simulink model "model"  (R2019b)
settings: Solver=VariableStepAuto  StartTime=0.0  StopTime=nb_time_unit_in_a_simulation/5  RelTol=1e-3
undefined symbols (not defined in the file or in its folder): air_mass_kg_rooms, Area_boiler, area_outdoor_rooms, Area_radiators, area_rooms_ground, area_walls_between_rooms, C_air, C_water, Energy_used_by_air_conditioner_for_1_timeunit_in_Watts_vector, Energy_used_by_air_mixer_for_1_timeunit_in_Watts, Energy_used_by_boiler_for_1_timeunit_in_Watts, initial_relative_humidity, initial_temp_water_in_boilers, initial_temperature_rooms, initial_temperature_water_in_radiator, k_boiler_border, k_radiators, k_wall_outdoor_rooms, k_walls_between_rooms, mass_water_radiator, matrix_AC_rooms_locations, matrix_boiler_radiator_connection, matrix_boiler_rooms_locations, matrix_radiator_rooms_locations, nb_air_cons, nb_boilers, nb_humans, nb_radiators, nb_rooms, nb_second_in_timeunit, outdoor_max_temp_A, outdoor_max_temp_B, outdoor_min_temp_A, outdoor_min_temp_B, tau_boiler, thickness_boiler, thickness_outdoor_rooms, thickness_radiator_pipes, thickness_walls_between_rooms, timeunit_in_a_day, Volume_radiators, Volume_rooms, water_weight_in_boiler, watt_generation_of_employe
libraries: dspmtrx3 x15, simulink x14
(part 2 of 2)

== system model/Physical model/Wall heat Exchange module/Value heat exchange outdoor -> rooms ==
  T_rooms : Inport
  outdoor : Inport  Port=2
  Gain : Gain  Gain=area_outdoor_rooms
  Gain1 : Gain  Gain=k_wall_outdoor_rooms
  Gain2 : Gain  Gain=ones(nb_rooms,1)./thickness_outdoor_rooms
  Sum : Sum  Inputs=|+-
  Q_outdoor_to_rooms : Outport
  wires:
  T_rooms/1 -> Sum/2
  outdoor/1 -> Sum/1
  Sum/1 -> Gain/1
  Gain/1 -> Gain1/1
  Gain1/1 -> Gain2/1
  Gain2/1 -> Q_outdoor_to_rooms/1

== system model/Physical model/Wall heat Exchange module/Value heat exchange within building ==
  "T_rooms " : Inport
  Constant : Constant  Value=diag(ones(nb_rooms,1))
  Gain3 : Gain  Gain=area_walls_between_rooms
  Gain4 : Gain  Gain=k_walls_between_rooms
  Gain8 : Gain  Gain=ones(nb_rooms,nb_rooms)./thickness_walls_between_rooms
  MATRIX WITH ROOM TEMPERATURE DIFFERENCE The area matrix after handles the case of non-adjacent rooms : dspmtrx3/Array-Vector Multiply  mode=Mute  saveAsFlag=0  Dimension=2  V_Source=Input port  V_VectFromMask=[0.5 0.25]  roundingMode=Floor  overflowMode=off  firstCoeffSignedness=Auto  firstCoeffDataTypeStr=Inherit: Same word length as input  firstCoeffMin=[]  firstCoeffMax=[]  firstCoeffLastDataTypeStr=Inherit: Same word length as input  prodOutputSignedness=Auto  accumSignedness=Auto  outputSignedness=Auto  outputDataTypeStr=Inherit: Same as product output  outputMin=[]  outputMax=[]  outputLastDataTypeStr=Inherit: Same as product output
      settings: SourceProductName=DSP System Toolbox  SourceProductBaseCode=DS
  Sum of Elements : Sum  Inputs=+  CollapseMode=Specified dimension  CollapseDim=2
  Q_in_building_to_rooms : Outport
  wires:
  Gain4/1 -> Gain8/1
  Gain3/1 -> Gain4/1
  MATRIX WITH ROOM TEMPERATURE DIFFERENCE The area matrix after handles the case of non-adjacent rooms/1 -> Gain3/1
  Gain8/1 -> Sum of Elements/1
  Sum of Elements/1 -> Q_in_building_to_rooms/1
  Constant/1 -> MATRIX WITH ROOM TEMPERATURE DIFFERENCE The area matrix after handles the case of non-adjacent rooms/1
  "T_rooms "/1 -> MATRIX WITH ROOM TEMPERATURE DIFFERENCE The area matrix after handles the case of non-adjacent rooms/2

== stateflow chart model/Controler module/HumidityController ==
  state ACLogic
    state ACOff
      en:acOn=0;
      state wet
      state norm
      state isWet(Humidity) [function]
        (default) -> (junction 24) : [Humidity>=upperbound]
      (default) -> norm
      norm -> wet : [isWet()]
    state ACOn1
      en:acOn=1;
    (default) -> ACOn1
    ACOn1 -> ACOff : after(40,sec)
        | [isDry(Humidity)]
    wet -> ACOn1 : after(40,sec)
        | [ACLogic.ACOn.isWet(Humidity)]
  state status = isDry(Humidity) [function]
    (default) -> (junction 16) : [Humidity<=lower_bound]
  data: Humidity function_input; Humidity function_input; status function_output; Humidity input; lower_bound input; upperbound input; acOn output
  events: sec input RISING_EDGE_EVENT

== stateflow chart model/Controler module/TemperatureController ==
  state ACLogic
    state ACOn
      en:acOn=1;
      state hot
      state norm
      state isHot(T_room) [function]
        (default) -> (junction 24) : [T_room>=upperbound]
      (default) -> norm
      norm -> hot : [isHot()]
    state ACOff
      en:acOn=0;
    (default) -> ACOff
    ACOff -> ACOn : after(40,sec)
        | [isCool(T_room)]
    hot -> ACOff : after(40,sec)
        | [ACLogic.ACOn.isHot(T_room)]
  state status = isCool(T_room) [function]
    (default) -> (junction 16) : [T_room<=lower_bound]
  data: T_room function_input; T_room function_input; status function_output; T_room input; lower_bound input; upperbound input; acOn output
  events: sec input RISING_EDGE_EVENT

== stateflow chart model/Controler module/Bang-Bang Controller ==
  state Heater [group]
    state Off
      entry: turn_boiler(OFF)
    state On
      en: turn_boiler(ON)
      (history)
      state HIGH
      state NORM
      state b = warm() [function]
        (default) -> (junction 41) : {b = !cold()}
      (default) -> HIGH
      HIGH -> NORM : [warm()]
    (default) -> Off
    On -> Off : after(20,sec)
    Off -> On : after(40,sec)
        | [cold()]
    NORM -> Off : [Heater.On.warm()]
  state turn_boiler(mode) [function]
    (default) -> (junction 32)
    (junction 32) -> (junction 33) [order 1] : [mode==ON]
    (junction 32) -> (junction 34) [order 2]
    (junction 33) -> (junction 34)
    (junction 34) -> (junction 36) : {boiler=mode}
  state b = cold() [function]
    (default) -> (junction 39) : { b = temp<=reference}
  data: b function_output boolean; mode function_input int8; b function_output boolean; boiler output int8; reference input fixdt(1,8,1,-15); OFF constant int8; ON constant int8 =1; temp input fixdt(1,8,0.390625,-15)
  events: sec input RISING_EDGE_EVENT
